simulink model "Solution_2"  (R2023b)
settings: Solver=VariableStepAuto  StartTime=0.0  StopTime=2  RelTol=1e-3
settings Model: Creator=ROG  LastModifiedBy=ROG

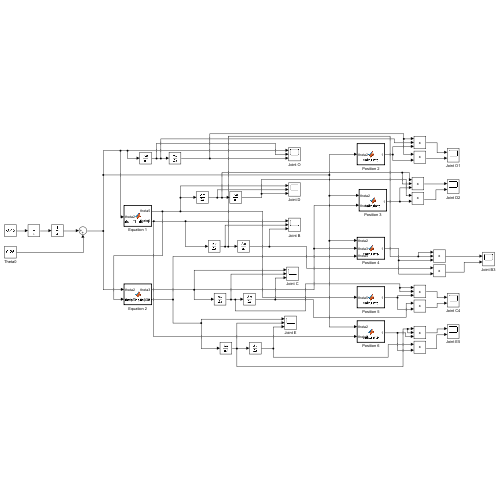
[thumbnail: Simulink's stored preview of the top-level diagram]
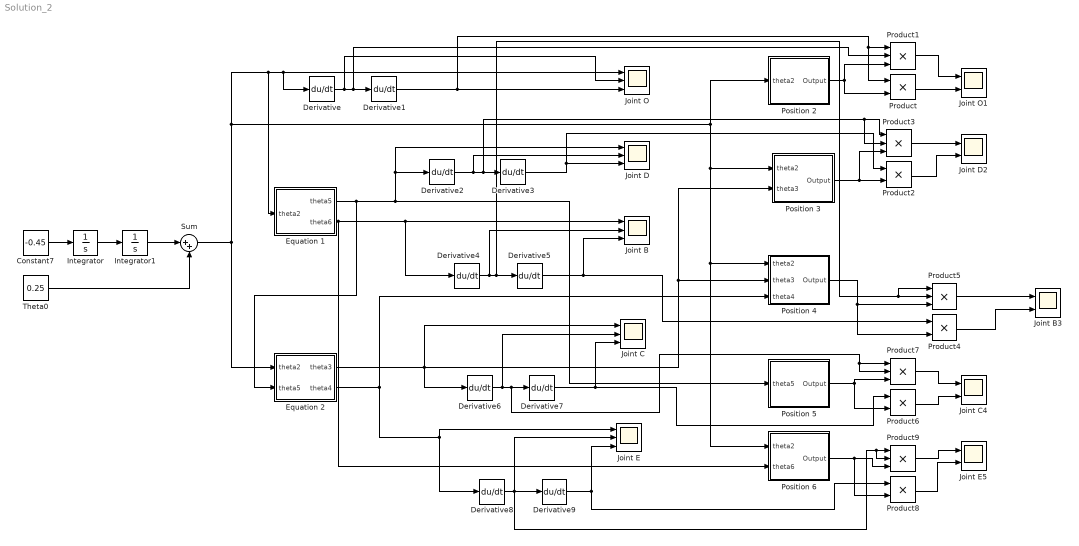
== system Solution_2 ==
  Constant7 : Constant  Value=-0.45
  Derivative{,1..9} (10 alike) : Derivative
  Equation 1 : MATLAB Function  TreatAsAtomicUnit=on
  Equation 2 : MATLAB Function  TreatAsAtomicUnit=on
  Integrator : Integrator
  Integrator1 : Integrator
  Joint B : Scope  NumInputPorts=3
  Joint B3 : Scope  NumInputPorts=2
  Joint C : Scope  NumInputPorts=3
  Joint C4 : Scope  NumInputPorts=2
  Joint D : Scope  NumInputPorts=3
  Joint D2 : Scope  NumInputPorts=2
  Joint E : Scope  NumInputPorts=3
  Joint E5 : Scope  NumInputPorts=2
  Joint O : Scope  NumInputPorts=3
  Joint O1 : Scope  NumInputPorts=2
  Position 2 : MATLAB Function  TreatAsAtomicUnit=on
  Position 3 : MATLAB Function  TreatAsAtomicUnit=on
  Position 4 : MATLAB Function  TreatAsAtomicUnit=on
  Position 5 : MATLAB Function  TreatAsAtomicUnit=on
  Position 6 : MATLAB Function  TreatAsAtomicUnit=on
  Product{,2,4,6,8} (5 alike) : Product
  Product{1,3,5,7,9} (5 alike) : Product  Inputs=3
  Sum : Sum  Inputs=|++
  Theta0 : Constant  Value=0.25
  wires:
  Constant7/1 -> Integrator/1
  Integrator/1 -> Integrator1/1
  Sum/1 -> Position 6/1(theta2), Position 4/1(theta2), Position 3/1(theta2), Position 2/1(theta2), Equation 1/1(theta2), Derivative/1, Joint O/1, Equation 2/1(theta2)
  Theta0/1 -> Sum/2
  Integrator1/1 -> Sum/1
  Derivative/1 -> Joint O/2, Product1/2, Derivative1/1
  Derivative1/1 -> Product1/1, Product/1, Joint O/3
  Derivative3/1 -> Product2/1, Joint D/3
  Derivative2/1 -> Joint D/2, Product3/2, Product3/1, Derivative3/1
  Equation 1/1(theta5) -> Equation 2/2(theta5), Position 5/1(theta5), Joint D/1, Derivative2/1
  Derivative5/1 -> Product4/1, Joint B/3
  Derivative4/1 -> Joint B/2, Product5/1, Product5/2, Derivative5/1
  Equation 1/2(theta6) -> Position 6/2(theta6), Joint B/1, Derivative4/1
  Derivative9/1 -> Joint E/3, Product8/1
  Derivative8/1 -> Product9/2, Product9/1, Joint E/2, Derivative9/1
  Derivative6/1 -> Joint C/2, Product7/1, Product7/2, Derivative7/1
  Equation 2/2(theta4) -> Joint E/1, Derivative8/1, Position 4/3(theta4)
  Equation 2/1(theta3) -> Position 4/2(theta3), Position 3/2(theta3), Derivative6/1, Joint C/1
  Derivative7/1 -> Product6/1, Joint C/3
  Position 2/1(Output) -> Product/2, Product1/3
  Product1/1 -> Joint O1/1
  Product/1 -> Joint O1/2
  Position 4/1(Output) -> Product4/2, Product5/3
  Position 5/1(Output) -> Product7/3, Product6/2
  Position 6/1(Output) -> Product8/2, Product9/3
  Product9/1 -> Joint E5/1
  Product8/1 -> Joint E5/2
  Product6/1 -> Joint C4/2
  Product7/1 -> Joint C4/1
  Position 3/1(Output) -> Product2/2, Product3/3
  Product3/1 -> Joint D2/1
  Product2/1 -> Joint D2/2
  Product5/1 -> Joint B3/1
  Product4/1 -> Joint B3/2

== matlab function Solution_2/Equation 2 ==
  data: theta2 input; theta3 output; theta4 output; theta5 input
function [theta3, theta4] = calculateTheta3Theta4(theta2, theta5)
    % Link Lengths
    L2 = 0.325;
    L3 = 0.16;
    L4 = 0.18;
    L5x = 0.1;
    L5y = 0.16;

    % Objective function to solve for theta3 and theta4
    objFunction = @(x) positionError2(x, L2, L3, L4, L5x, L5y, theta2, theta5);

    % Initial guess
    initialGuess = [0, 0];

    % Options for fsolve
    options = optimoptions('fsolve', 'Algorithm', 'levenberg-marquardt');

    % Solve using fsolve
    solution = fsolve(objFunction, initialGuess, options);

    % Extract the solutions
    theta3 = solution(1);
    theta4 = solution(2);
end

function error = positionError2(x, L2, L3, L4, L5x, L5y, theta2, theta5)
    % Compute the error between the target and actual positions
    End = [0.62; 0.19];
    target = Position(L2, theta2) + Position(L3, x(1)) + Position(L4, x(2)) - Position(L5x, theta5) - Position(L5y, (theta5 - pi/2));
    error = target - End;
end

function pos = Position(L, theta)
    % Compute the position vector
    pos = [L * cos(theta); L * sin(theta)];
end

== matlab function Solution_2/Equation 1 ==
  data: theta2 input; theta5 output; theta6 output
function [theta5, theta6] = calculateTheta5Theta6(theta2)
    % Link Lengths  
    L2 = 0.325; 

    % Objective function to solve for theta5 and theta6
    objFunction = @(x) positionError(x, L2, theta2);

    % Initial guess
    initialGuess = [0, 0];

    % Options for fsolve
    options = optimoptions('fsolve', 'Algorithm', 'levenberg-marquardt');

    % Solve using fsolve
    solution = fsolve(objFunction, initialGuess, options);

    % Extract the solutions
    theta5 = solution(1);
    theta6 = solution(2);
end

function error = positionError(x, L2, theta2)
    % Compute the error between the target and actual positions
    L6 = 0.35;
    End = [0.62; 0.19];
    target = Position(L2 - 0.08, theta2) + Position(L6, x(2)) - Position(0.1, x(1)) - Position(0.08, x(1) - pi/2);
    error = target - End;
end

function pos = Position(L, theta)
    % Compute the position vector
    pos = [L * cos(theta); L * sin(theta)];
end

== matlab function Solution_2/Position 2 ==
  data: Output output; theta2 input
function Output  = calculate(theta2)
L1x = 0.62; 
L1y = 0.19; 
L2 = 0.325; 
L3 = 0.16; 
L4 = 0.18; 
L5x = 0.1; 
L5y = 0.16; 
L6 = 0.35;

lg2 = 0.17115; 
lg3 = 0.09026; 
lg4 = 0.09; 
lg6 = 0.175;
Output =Position(lg2, theta2);
end
function pos = Position(L, theta)
    % Compute the position vector
    pos = [L * cos(theta); L * sin(theta)];
end

== matlab function Solution_2/Position 3 ==
  data: theta2 input; Output output; theta3 input
function Output = calculate(theta2,theta3)
L1x = 0.62; 
L1y = 0.19; 
L2 = 0.325; 
L3 = 0.16; 
L4 = 0.18; 
L5x = 0.1; 
L5y = 0.16; 
L6 = 0.35;

lg2 = 0.17115; 
lg3 = 0.09026; 
lg4 = 0.09; 
lg6 = 0.175;
Output = Position(L2, theta2) + Position(lg3, theta3);
end
function pos = Position(L, theta)
    % Compute the position vector
    pos = [L * cos(theta); L * sin(theta)];
end

== matlab function Solution_2/Position 4 ==
  data: theta2 input; Output output; theta3 input; theta4 input
function Output = calculate(theta2,theta3,theta4)
L1x = 0.62; 
L1y = 0.19; 
L2 = 0.325; 
L3 = 0.16; 
L4 = 0.18; 
L5x = 0.1; 
L5y = 0.16; 
L6 = 0.35;

lg2 = 0.17115; 
lg3 = 0.09026; 
lg4 = 0.09; 
lg6 = 0.175;
Output = Position(L2, theta2) + Position(L3, theta3) + Position(lg4, theta4);
end
function pos = Position(L, theta)
    % Compute the position vector
    pos = [L * cos(theta); L * sin(theta)];
end

== matlab function Solution_2/Position 5 ==
  data: theta5 input; Output output
function Output = calculate(theta5)
L1x = 0.62; 
L1y = 0.19; 
L2 = 0.325; 
L3 = 0.16; 
L4 = 0.18; 
L5x = 0.1; 
L5y = 0.16; 
L6 = 0.35;

lg2 = 0.17115; 
lg3 = 0.09026; 
lg4 = 0.09; 
lg6 = 0.175;
Output =Position(L5x+0.02-0.0436, theta5) - Position(0.0754-0.02, (theta5 - pi/2));
end
function pos = Position(L, theta)
    % Compute the position vector
    pos = [L * cos(theta); L * sin(theta)];
end

== matlab function Solution_2/Position 6 ==
  data: theta2 input; Output output; theta6 input
function Output = calculate(theta2,theta6)
L1x = 0.62; 
L1y = 0.19; 
L2 = 0.325; 
L3 = 0.16; 
L4 = 0.18; 
L5x = 0.1; 
L5y = 0.16; 
L6 = 0.35;

lg2 = 0.17115; 
lg3 = 0.09026; 
lg4 = 0.09; 
lg6 = 0.175;
Output = Position((L2-0.08), theta2) + Position(lg6, theta6);
end
function pos = Position(L, theta)
    % Compute the position vector
    pos = [L * cos(theta); L * sin(theta)];
end
